simulink model "gm_qft_3qubit_fixpt"  (R2024b)
settings: Solver=VariableStepAuto  StartTime=0.0  StopTime=10.0  RelTol=1e-3
settings Model: SimulationMode=accelerator  Creator=bonga  LastModifiedBy=bonga
settings DebuggingCC: InheritedTsInSrcMsg=none

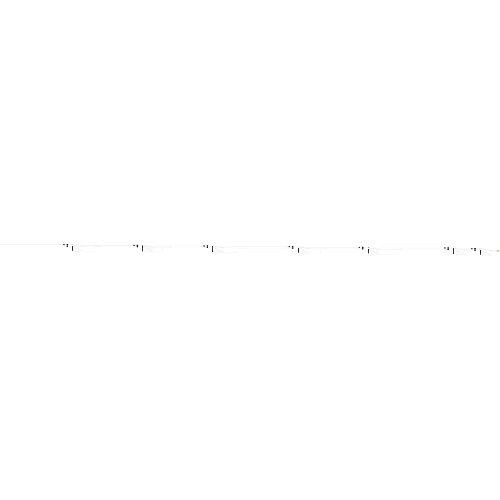
[thumbnail: Simulink's stored preview of the top-level diagram]
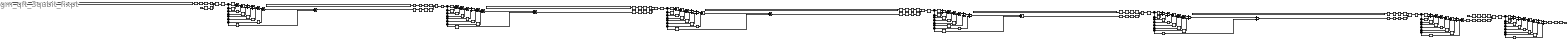
== system gm_qft_3qubit_fixpt ==
  initial_state : Inport  OutDataTypeStr=fixdt(0,1,0,'DataTypeOverride', 'Off')  PortDimensions=[8 1]  SampleTime=1
  MMul_add_01 : Sum  OutDataTypeStr=fixdt(1, 18, 14)  SampleTime=1
  MMul_add_011 : Sum  OutDataTypeStr=fixdt(1, 32, 26)  SampleTime=1
  MMul_add_012 : Sum  OutDataTypeStr=fixdt(1, 19, 13)  SampleTime=1
  MMul_add_013 : Sum  OutDataTypeStr=fixdt(1, 32, 26)  SampleTime=1
  MMul_add_014 : Sum  OutDataTypeStr=fixdt(1, 19, 13)  SampleTime=1
  MMul_add_015 : Sum  OutDataTypeStr=fixdt(1, 19, 13)  SampleTime=1
  MMul_add_016 : Sum  OutDataTypeStr=fixdt(1, 18, 13)  SampleTime=1
  MMul_add_{12,23,34,45,56,67} (6 alike) : Sum  OutDataTypeStr=fixdt(1, 18, 14)  SampleTime=1
  MMul_add_{121,123,231,233,341,343,451,453,561,563,671,673} (12 alike) : Sum  OutDataTypeStr=fixdt(1, 32, 26)  SampleTime=1
  MMul_add_{122,124..125,232,234..235,342,344..345,452,454..455,562,564..565,672,674..675} (18 alike) : Sum  OutDataTypeStr=fixdt(1, 19, 13)  SampleTime=1
  MMul_add_{126,236,346,456,566,676} (6 alike) : Sum  OutDataTypeStr=fixdt(1, 18, 13)  SampleTime=1
  MMul_dot_product : Product  Inputs=**  OutDataTypeStr=fixdt(1, 18, 14)  SampleTime=1
  MMul_dot_product1 : Product  Inputs=**  OutDataTypeStr=fixdt(1, 32, 26)  SampleTime=1
  MMul_dot_product2 : Product  Inputs=**  OutDataTypeStr=fixdt(1, 19, 13)  SampleTime=1
  MMul_dot_product3 : Product  Inputs=**  OutDataTypeStr=fixdt(1, 32, 26)  SampleTime=1
  MMul_dot_product4 : Product  Inputs=**  OutDataTypeStr=fixdt(1, 19, 13)  SampleTime=1
  MMul_dot_product5 : Product  Inputs=**  OutDataTypeStr=fixdt(1, 19, 13)  SampleTime=1
  MMul_dot_product6 : Product  Inputs=**  OutDataTypeStr=fixdt(1, 18, 13)  SampleTime=1
  Row2Col_in{0..1,11..16} (8 alike) : Reshape  OutputDimensionality=Column vector (2-D)
  Row2Col_in01 : Reshape  OutputDimensionality=Column vector (2-D)
  Row2Col_in02 : Reshape  OutputDimensionality=Column vector (2-D)
  Row2Col_in03 : Reshape  OutputDimensionality=Column vector (2-D)
  Row2Col_in04 : Reshape  OutputDimensionality=Column vector (2-D)
  Row2Col_in05 : Reshape  OutputDimensionality=Column vector (2-D)
  Row2Col_in06 : Reshape  OutputDimensionality=Column vector (2-D)
  dtc : DataTypeConversion  OutDataTypeStr=fixdt(1, 14, 14)  SampleTime=1  SaturateOnIntegerOverflow=off  RndMeth=Floor
  dtc1 : DataTypeConversion  OutDataTypeStr=fixdt(1, 14, 14)  SampleTime=1  SaturateOnIntegerOverflow=off  RndMeth=Floor
  dtc{2..7} (6 alike) : DataTypeConversion  OutDataTypeStr=fixdt(1, 14, 13)  SampleTime=1  SaturateOnIntegerOverflow=off  RndMeth=Floor
  final_state_reg : Delay  DelayLength=double(1)  InitialCondition=0  SampleTime=1
  gain_const : Constant  Value=[1;0;0;0;0;0;0;0;0;1;0;0;0;0;0;0;0;0;1;0;0;0;0;0;0;0;0;1;0;0;0;0;0;0;0;0;1;0;0;0;0;0;0;0;0;1;0;0;0;0;0;0;0;0;1;0;0;0;0;0;0;0;0;1]  OutDataTypeStr=fixdt(0, 1, 0)  SampleTime=1
  gain_const1 : Constant  Value="complex(fi(\"numerictype\",numerictype(1,14,13),\"fimath\",fimath(\"RoundingMethod\", \"Floor\",\"OverflowAction\", \"Wrap\",\"ProductMode\",\"FullPrecision\",\"SumMode\",\"FullPrecision\"),\"Value\",\"[0.70703125;0.70703125;0;0;0;0;0;0;0.70703125;-0.7071533203125;0;0;0;0;0;0;0;0;0.70703125;0.70703125;0;0;0;0;0;0;0.70703125;-0.7071533203125;0;0;0;0;0;0;0;0;0.70703125;0.70703125;0;0;0;0;0;0;0.70703125;-0.7071533203125;0;0;0;0;0;0;0;0;0.70703125;0.70703125;0;0;0;0;0;0;0.70703125;-0.7071533203125]\"), fi(\"numerictype\",numerictype(1,14,13),\"fimath\",fimath(\"RoundingMethod\", \"Floor\",\"OverflowAction\", \"Wrap\",\"ProductMode\",\"FullPrecision\",\"SumMode\",\"FullPrecision\"),\"Value\",\"[0;0;0;0;0;0;0;0;0;0;0;0;0;0;0;0;0;0;0;0;0;0;0;0;0;0;0;0;0;0;0;0;0;0;0;0;0;0;0;0;0;0;0;0;0;0;0;0;0;0;0;0;0;0;0;0;0;0;0;0;0;0;0;0]\"))"  OutDataTypeStr=fixdt(1, 14, 13)  SampleTime=1
  gain_const2 : Constant  Value="complex(fi(\"numerictype\",numerictype(0,1,0),\"fimath\",fimath(\"RoundingMethod\", \"Floor\",\"OverflowAction\", \"Wrap\",\"ProductMode\",\"FullPrecision\",\"SumMode\",\"FullPrecision\"),\"Value\",\"[1;0;0;0;0;0;0;0;0;1;0;0;0;0;0;0;0;0;1;0;0;0;0;0;0;0;0;1;0;0;0;0;0;0;0;0;1;0;0;0;0;0;0;0;0;1;0;0;0;0;0;0;0;0;1;0;0;0;0;0;0;0;0;1]\"), fi(\"numerictype\",numerictype(0,1,0),\"fimath\",fimath(\"RoundingMethod\", \"Floor\",\"OverflowAction\", \"Wrap\",\"ProductMode\",\"FullPrecision\",\"SumMode\",\"FullPrecision\"),\"Value\",\"[0;0;0;0;0;0;0;0;0;0;0;0;0;0;0;0;0;0;0;0;0;0;0;0;0;0;0;0;0;0;0;0;0;0;0;0;0;0;0;0;0;0;0;0;0;0;0;0;0;0;0;0;0;0;0;0;0;0;0;0;0;0;0;0]\"))"  OutDataTypeStr=fixdt(0, 1, 0)  SampleTime=1
  gain_const3 : Constant  Value="complex(fi(\"numerictype\",numerictype(1,14,13),\"fimath\",fimath(\"RoundingMethod\", \"Floor\",\"OverflowAction\", \"Wrap\",\"ProductMode\",\"FullPrecision\",\"SumMode\",\"FullPrecision\"),\"Value\",\"[0.70703125;0;0.70703125;0;0;0;0;0;0;0.70703125;0;0.70703125;0;0;0;0;0.70703125;0;-0.707275390625;0;0;0;0;0;0;0.70703125;0;-0.707275390625;0;0;0;0;0;0;0;0;0.70703125;0;0.70703125;0;0;0;0;0;0;0.70703125;0;0.70703125;0;0;0;0;0.70703125;0;-0.707275390625;0;0;0;0;0;0;0.70703125;0;-0.707275390625]\"), fi(\"numerictype\",numerictype(1,14,13),\"fimath\",fimath(\"RoundingMethod\", \"Floor\",\"OverflowAction\", \"Wrap\",\"ProductMode\",\"FullPrecision\",\"SumMode\",\"FullPrecision\"),\"Value\",\"[0;0;0;0;0;0;0;0;0;0;0;0;0;0;0;0;0;0;0;0;0;0;0;0;0;0;0;0;0;0;0;0;0;0;0;0;0;0;0;0;0;0;0;0;0;0;0;0;0;0;0;0;0;0;0;0;0;0;0;0;0;0;0;0]\"))"  OutDataTypeStr=fixdt(1, 14, 13)  SampleTime=1
  gain_const4 : Constant  Value="complex(fi(\"numerictype\",numerictype(0,1,0),\"fimath\",fimath(\"RoundingMethod\", \"Floor\",\"OverflowAction\", \"Wrap\",\"ProductMode\",\"FullPrecision\",\"SumMode\",\"FullPrecision\"),\"Value\",\"[1;0;0;0;0;0;0;0;0;1;0;0;0;0;0;0;0;0;1;0;0;0;0;0;0;0;0;1;0;0;0;0;0;0;0;0;1;0;0;0;0;0;0;0;0;1;0;0;0;0;0;0;0;0;1;0;0;0;0;0;0;0;0;1]\"), fi(\"numerictype\",numerictype(0,1,0),\"fimath\",fimath(\"RoundingMethod\", \"Floor\",\"OverflowAction\", \"Wrap\",\"ProductMode\",\"FullPrecision\",\"SumMode\",\"FullPrecision\"),\"Value\",\"[0;0;0;0;0;0;0;0;0;0;0;0;0;0;0;0;0;0;0;0;0;0;0;0;0;0;0;0;0;0;0;0;0;0;0;0;0;0;0;0;0;0;0;0;0;0;0;0;0;0;0;0;0;0;0;0;0;0;0;0;0;0;0;0]\"))"  OutDataTypeStr=fixdt(0, 1, 0)  SampleTime=1
  gain_const5 : Constant  Value="complex(fi(\"numerictype\",numerictype(0,1,0),\"fimath\",fimath(\"RoundingMethod\", \"Floor\",\"OverflowAction\", \"Wrap\",\"ProductMode\",\"FullPrecision\",\"SumMode\",\"FullPrecision\"),\"Value\",\"[1;0;0;0;0;0;0;0;0;1;0;0;0;0;0;0;0;0;1;0;0;0;0;0;0;0;0;1;0;0;0;0;0;0;0;0;1;0;0;0;0;0;0;0;0;1;0;0;0;0;0;0;0;0;1;0;0;0;0;0;0;0;0;1]\"), fi(\"numerictype\",numerictype(0,1,0),\"fimath\",fimath(\"RoundingMethod\", \"Floor\",\"OverflowAction\", \"Wrap\",\"ProductMode\",\"FullPrecision\",\"SumMode\",\"FullPrecision\"),\"Value\",\"[0;0;0;0;0;0;0;0;0;0;0;0;0;0;0;0;0;0;0;0;0;0;0;0;0;0;0;0;0;0;0;0;0;0;0;0;0;0;0;0;0;0;0;0;0;0;0;0;0;0;0;0;0;0;0;0;0;0;0;0;0;0;0;0]\"))"  OutDataTypeStr=fixdt(0, 1, 0)  SampleTime=1
  gain_const6 : Constant  Value="complex(fi(\"numerictype\",numerictype(1,14,13),\"fimath\",fimath(\"RoundingMethod\", \"Floor\",\"OverflowAction\", \"Wrap\",\"ProductMode\",\"FullPrecision\",\"SumMode\",\"FullPrecision\"),\"Value\",\"[0.70703125;0;0;0;0.70703125;0;0;0;0;0.70703125;0;0;0;0.70703125;0;0;0;0;0.70703125;0;0;0;0.70703125;0;0;0;0;0.70703125;0;0;0;0.70703125;0.70703125;0;0;0;-0.707275390625;0;0;0;0;0.70703125;0;0;0;-0.707275390625;0;0;0;0;0.70703125;0;0;0;-0.707275390625;0;0;0;0;0.70703125;0;0;0;-0.707275390625]\"), fi(\"numerictype\",numerictype(1,14,13),\"fimath\",fimath(\"RoundingMethod\", \"Floor\",\"OverflowAction\", \"Wrap\",\"ProductMode\",\"FullPrecision\",\"SumMode\",\"FullPrecision\"),\"Value\",\"[0;0;0;0;0;0;0;0;0;0;0;0;0;0;0;0;0;0;0;0;0;0;0;0;0;0;0;0;0;0;0;0;0;0;0;0;0;0;0;0;0;0;0;0;0;0;0;0;0;0;0;0;0;0;0;0;0;0;0;0;0;0;0;0]\"))"  OutDataTypeStr=fixdt(1, 14, 13)  SampleTime=1
  reshape_dotProduct{,1..6} (7 alike) : Reshape  OutputDimensionality=Customize  OutputDimensions=[8,8]
  reshape_mmulResult{,1..6} (7 alike) : Reshape  OutputDimensionality=Customize  OutputDimensions=[8,1]
  select_0 : Selector  NumberOfDimensions=2  IndexOptions=Index vector (dialog),Select all  Indices=double(1),[]  OutputSizes=1
  select_01 : Selector  NumberOfDimensions=2  IndexOptions=Index vector (dialog),Select all  Indices=double(1),[]  OutputSizes=1
  select_02 : Selector  NumberOfDimensions=2  IndexOptions=Index vector (dialog),Select all  Indices=double(1),[]  OutputSizes=1
  select_03 : Selector  NumberOfDimensions=2  IndexOptions=Index vector (dialog),Select all  Indices=double(1),[]  OutputSizes=1
  select_04 : Selector  NumberOfDimensions=2  IndexOptions=Index vector (dialog),Select all  Indices=double(1),[]  OutputSizes=1
  select_05 : Selector  NumberOfDimensions=2  IndexOptions=Index vector (dialog),Select all  Indices=double(1),[]  OutputSizes=1
  select_06 : Selector  NumberOfDimensions=2  IndexOptions=Index vector (dialog),Select all  Indices=double(1),[]  OutputSizes=1
  select_{1,11..16} (7 alike) : Selector  NumberOfDimensions=2  IndexOptions=Index vector (dialog),Select all  Indices=double(2),[]  OutputSizes=1
  select_{2,21..26} (7 alike) : Selector  NumberOfDimensions=2  IndexOptions=Index vector (dialog),Select all  Indices=double(3),[]  OutputSizes=1
  select_{3,31..36} (7 alike) : Selector  NumberOfDimensions=2  IndexOptions=Index vector (dialog),Select all  Indices=double(4),[]  OutputSizes=1
  select_{4,41..46} (7 alike) : Selector  NumberOfDimensions=2  IndexOptions=Index vector (dialog),Select all  Indices=double(5),[]  OutputSizes=1
  select_{5,51..56} (7 alike) : Selector  NumberOfDimensions=2  IndexOptions=Index vector (dialog),Select all  Indices=double(6),[]  OutputSizes=1
  select_{6,61..66} (7 alike) : Selector  NumberOfDimensions=2  IndexOptions=Index vector (dialog),Select all  Indices=double(7),[]  OutputSizes=1
  select_{7,71..76} (7 alike) : Selector  NumberOfDimensions=2  IndexOptions=Index vector (dialog),Select all  Indices=double(8),[]  OutputSizes=1
  select_indices0 : Selector  InputPortWidth=64  IndexOptions=Index vector (dialog)  Indices=double([1 9 17 25 33 41 49 57 2 10 18 26 34 42 50 58 3 11 19 27 35 43 51 59 4 12 20 28 36 44 52 60 5 13 21 29 37 45 53 61 6 14 22 30 38 46 54 62 7 15 23 31 39 47 55 63 8 16 24 32 40 48 56 64])  OutputSizes=1
  select_indices01 : Selector  InputPortWidth=64  IndexOptions=Index vector (dialog)  Indices=double([1 9 17 25 33 41 49 57 2 10 18 26 34 42 50 58 3 11 19 27 35 43 51 59 4 12 20 28 36 44 52 60 5 13 21 29 37 45 53 61 6 14 22 30 38 46 54 62 7 15 23 31 39 47 55 63 8 16 24 32 40 48 56 64])  OutputSizes=1
  select_indices02 : Selector  InputPortWidth=64  IndexOptions=Index vector (dialog)  Indices=double([1 9 17 25 33 41 49 57 2 10 18 26 34 42 50 58 3 11 19 27 35 43 51 59 4 12 20 28 36 44 52 60 5 13 21 29 37 45 53 61 6 14 22 30 38 46 54 62 7 15 23 31 39 47 55 63 8 16 24 32 40 48 56 64])  OutputSizes=1
  select_indices03 : Selector  InputPortWidth=64  IndexOptions=Index vector (dialog)  Indices=double([1 9 17 25 33 41 49 57 2 10 18 26 34 42 50 58 3 11 19 27 35 43 51 59 4 12 20 28 36 44 52 60 5 13 21 29 37 45 53 61 6 14 22 30 38 46 54 62 7 15 23 31 39 47 55 63 8 16 24 32 40 48 56 64])  OutputSizes=1
  select_indices04 : Selector  InputPortWidth=64  IndexOptions=Index vector (dialog)  Indices=double([1 9 17 25 33 41 49 57 2 10 18 26 34 42 50 58 3 11 19 27 35 43 51 59 4 12 20 28 36 44 52 60 5 13 21 29 37 45 53 61 6 14 22 30 38 46 54 62 7 15 23 31 39 47 55 63 8 16 24 32 40 48 56 64])  OutputSizes=1
  select_indices05 : Selector  InputPortWidth=64  IndexOptions=Index vector (dialog)  Indices=double([1 9 17 25 33 41 49 57 2 10 18 26 34 42 50 58 3 11 19 27 35 43 51 59 4 12 20 28 36 44 52 60 5 13 21 29 37 45 53 61 6 14 22 30 38 46 54 62 7 15 23 31 39 47 55 63 8 16 24 32 40 48 56 64])  OutputSizes=1
  select_indices06 : Selector  InputPortWidth=64  IndexOptions=Index vector (dialog)  Indices=double([1 9 17 25 33 41 49 57 2 10 18 26 34 42 50 58 3 11 19 27 35 43 51 59 4 12 20 28 36 44 52 60 5 13 21 29 37 45 53 61 6 14 22 30 38 46 54 62 7 15 23 31 39 47 55 63 8 16 24 32 40 48 56 64])  OutputSizes=1
  select_indices{1,11..16} (7 alike) : Selector  InputPortWidth=8  IndexOptions=Index vector (dialog)  Indices=double([1 2 3 4 5 6 7 8 1 2 3 4 5 6 7 8 1 2 3 4 5 6 7 8 1 2 3 4 5 6 7 8 1 2 3 4 5 6 7 8 1 2 3 4 5 6 7 8 1 2 3 4 5 6 7 8 1 2 3 4 5 6 7 8])  OutputSizes=1
  t{,1..6} (7 alike) : Reshape  OutputDimensionality=Customize  OutputDimensions=[8,8]
  vectorized_in0 : Reshape  OutputDimensionality=Row vector (2-D)
  vectorized_in01 : Reshape  OutputDimensionality=Row vector (2-D)
  vectorized_in02 : Reshape  OutputDimensionality=Row vector (2-D)
  vectorized_in03 : Reshape  OutputDimensionality=Row vector (2-D)
  vectorized_in04 : Reshape  OutputDimensionality=Row vector (2-D)
  vectorized_in05 : Reshape  OutputDimensionality=Row vector (2-D)
  vectorized_in06 : Reshape  OutputDimensionality=Row vector (2-D)
  final_state : Outport  OutDataTypeStr=fixdt(1,14,14,'DataTypeOverride', 'Off')  PortDimensions=[8 1]  SampleTime=1
      settings: SignalType=complex
  wires:
  select_indices0/1 -> Row2Col_in0/1
  dtc2/1 -> dtc1/1
  gain_const4/1 -> t4/1
  select_01/1 -> MMul_add_011/1
  reshape_mmulResult1/1 -> dtc2/1
  select_0/1 -> MMul_add_01/1
  MMul_add_561/1 -> MMul_add_671/1
  reshape_mmulResult2/1 -> dtc3/1
  reshape_mmulResult3/1 -> dtc4/1
  dtc6/1 -> select_indices14/1
  select_indices01/1 -> Row2Col_in01/1
  reshape_mmulResult5/1 -> dtc6/1
  dtc7/1 -> select_indices15/1
  select_indices1/1 -> Row2Col_in1/1
  vectorized_in0/1 -> select_indices0/1
  Row2Col_in0/1 -> MMul_dot_product/1
  MMul_dot_product/1 -> reshape_dotProduct/1
  select_12/1 -> MMul_add_012/2
  MMul_add_12/1 -> MMul_add_23/1
  select_4/1 -> MMul_add_34/2
  select_5/1 -> MMul_add_45/2
  select_53/1 -> MMul_add_453/2
  t1/1 -> vectorized_in01/1
  MMul_add_011/1 -> MMul_add_121/1
  MMul_add_673/1 -> reshape_mmulResult3/1
  MMul_add_234/1 -> MMul_add_344/1
  MMul_add_344/1 -> MMul_add_454/1
  t5/1 -> vectorized_in05/1
  MMul_add_564/1 -> MMul_add_674/1
  MMul_add_34/1 -> MMul_add_45/1
  select_11/1 -> MMul_add_011/2
  select_15/1 -> MMul_add_015/2
  select_16/1 -> MMul_add_016/2
  select_54/1 -> MMul_add_454/2
  select_63/1 -> MMul_add_563/2
  MMul_add_015/1 -> MMul_add_125/1
  select_64/1 -> MMul_add_564/2
  select_24/1 -> MMul_add_124/2
  MMul_add_235/1 -> MMul_add_345/1
  MMul_add_236/1 -> MMul_add_346/1
  MMul_add_125/1 -> MMul_add_235/1
  gain_const3/1 -> t3/1
  select_43/1 -> MMul_add_343/2
  MMul_add_676/1 -> reshape_mmulResult6/1
  select_26/1 -> MMul_add_126/2
  select_indices14/1 -> Row2Col_in14/1
  gain_const2/1 -> t2/1
  vectorized_in03/1 -> select_indices03/1
  MMul_add_121/1 -> MMul_add_231/1
  reshape_dotProduct6/1 -> select_76/1, select_66/1, select_56/1, select_46/1, select_36/1, select_26/1, select_16/1, select_06/1
  reshape_mmulResult4/1 -> dtc5/1
  reshape_dotProduct4/1 -> select_74/1, select_64/1, select_54/1, select_44/1, select_34/1, select_24/1, select_14/1, select_04/1
  select_indices13/1 -> Row2Col_in13/1
  select_indices11/1 -> Row2Col_in11/1
  select_14/1 -> MMul_add_014/2
  select_21/1 -> MMul_add_121/2
  MMul_add_671/1 -> reshape_mmulResult1/1
  MMul_dot_product1/1 -> reshape_dotProduct1/1
  select_04/1 -> MMul_add_014/1
  Row2Col_in13/1 -> MMul_dot_product3/2
  select_73/1 -> MMul_add_673/2
  select_indices16/1 -> Row2Col_in16/1
  dtc4/1 -> select_indices12/1
  select_06/1 -> MMul_add_016/1
  select_75/1 -> MMul_add_675/2
  Row2Col_in03/1 -> MMul_dot_product3/1
  select_indices04/1 -> Row2Col_in04/1
  MMul_add_122/1 -> MMul_add_232/1
  select_7/1 -> MMul_add_67/2
  MMul_add_123/1 -> MMul_add_233/1
  MMul_add_231/1 -> MMul_add_341/1
  select_42/1 -> MMul_add_342/2
  Row2Col_in15/1 -> MMul_dot_product5/2
  reshape_dotProduct2/1 -> select_62/1, select_72/1, select_52/1, select_42/1, select_32/1, select_22/1, select_12/1, select_02/1
  select_02/1 -> MMul_add_012/1
  select_62/1 -> MMul_add_562/2
  gain_const6/1 -> t6/1
  select_indices06/1 -> Row2Col_in06/1
  vectorized_in05/1 -> select_indices05/1
  t4/1 -> vectorized_in04/1
  MMul_add_342/1 -> MMul_add_452/1
  t3/1 -> vectorized_in03/1
  MMul_dot_product4/1 -> reshape_dotProduct4/1
  vectorized_in02/1 -> select_indices02/1
  select_41/1 -> MMul_add_341/2
  Row2Col_in01/1 -> MMul_dot_product1/1
  select_22/1 -> MMul_add_122/2
  select_34/1 -> MMul_add_234/2
  Row2Col_in12/1 -> MMul_dot_product2/2
  MMul_add_343/1 -> MMul_add_453/1
  MMul_add_562/1 -> MMul_add_672/1
  t/1 -> vectorized_in0/1
  MMul_add_01/1 -> MMul_add_12/1
  vectorized_in01/1 -> select_indices01/1
  select_03/1 -> MMul_add_013/1
  select_32/1 -> MMul_add_232/2
  MMul_add_233/1 -> MMul_add_343/1
  select_2/1 -> MMul_add_12/2
  MMul_add_453/1 -> MMul_add_563/1
  dtc5/1 -> select_indices13/1
  MMul_add_346/1 -> MMul_add_456/1
  MMul_dot_product3/1 -> reshape_dotProduct3/1
  reshape_dotProduct1/1 -> select_71/1, select_61/1, select_51/1, select_41/1, select_31/1, select_21/1, select_11/1, select_01/1
  MMul_add_23/1 -> MMul_add_34/1
  gain_const5/1 -> t5/1
  gain_const1/1 -> t1/1
  MMul_add_452/1 -> MMul_add_562/1
  select_72/1 -> MMul_add_672/2
  select_46/1 -> MMul_add_346/2
  MMul_add_451/1 -> MMul_add_561/1
  Row2Col_in04/1 -> MMul_dot_product4/1
  select_61/1 -> MMul_add_561/2
  MMul_add_232/1 -> MMul_add_342/1
  reshape_mmulResult/1 -> dtc/1
  vectorized_in04/1 -> select_indices04/1
  select_05/1 -> MMul_add_015/1
  MMul_add_013/1 -> MMul_add_123/1
  select_45/1 -> MMul_add_345/2
  select_66/1 -> MMul_add_566/2
  select_13/1 -> MMul_add_013/2
  dtc1/1 -> select_indices1/1
  MMul_add_563/1 -> MMul_add_673/1
  Row2Col_in05/1 -> MMul_dot_product5/1
  select_44/1 -> MMul_add_344/2
  Row2Col_in11/1 -> MMul_dot_product1/2
  MMul_add_675/1 -> reshape_mmulResult5/1
  dtc3/1 -> select_indices11/1
  MMul_dot_product2/1 -> reshape_dotProduct2/1
  select_74/1 -> MMul_add_674/2
  select_33/1 -> MMul_add_233/2
  t2/1 -> vectorized_in02/1
  MMul_add_124/1 -> MMul_add_234/1
  Row2Col_in14/1 -> MMul_dot_product4/2
  Row2Col_in16/1 -> MMul_dot_product6/2
  MMul_add_456/1 -> MMul_add_566/1
  select_indices12/1 -> Row2Col_in12/1
  MMul_add_674/1 -> reshape_mmulResult4/1
  select_indices02/1 -> Row2Col_in02/1
  select_indices03/1 -> Row2Col_in03/1
  MMul_dot_product5/1 -> reshape_dotProduct5/1
  reshape_mmulResult6/1 -> dtc7/1
  select_31/1 -> MMul_add_231/2
  MMul_add_341/1 -> MMul_add_451/1
  MMul_dot_product6/1 -> reshape_dotProduct6/1
  select_52/1 -> MMul_add_452/2
  MMul_add_016/1 -> MMul_add_126/1
  select_76/1 -> MMul_add_676/2
  reshape_dotProduct5/1 -> select_65/1, select_75/1, select_55/1, select_45/1, select_35/1, select_25/1, select_15/1, select_05/1
  MMul_add_012/1 -> MMul_add_122/1
  select_6/1 -> MMul_add_56/2
  t6/1 -> vectorized_in06/1
  MMul_add_566/1 -> MMul_add_676/1
  Row2Col_in02/1 -> MMul_dot_product2/1
  MMul_add_565/1 -> MMul_add_675/1
  select_3/1 -> MMul_add_23/2
  MMul_add_454/1 -> MMul_add_564/1
  dtc/1 -> final_state_reg/1
  MMul_add_45/1 -> MMul_add_56/1
  select_56/1 -> MMul_add_456/2
  select_35/1 -> MMul_add_235/2
  final_state_reg/1 -> final_state/1
  select_25/1 -> MMul_add_125/2
  MMul_add_672/1 -> reshape_mmulResult2/1
  Row2Col_in1/1 -> MMul_dot_product/2
  MMul_add_014/1 -> MMul_add_124/1
  reshape_dotProduct/1 -> select_7/1, select_6/1, select_5/1, select_4/1, select_3/1, select_2/1, select_1/1, select_0/1
  MMul_add_67/1 -> reshape_mmulResult/1
  vectorized_in06/1 -> select_indices06/1
  select_23/1 -> MMul_add_123/2
  Row2Col_in06/1 -> MMul_dot_product6/1
  MMul_add_56/1 -> MMul_add_67/1
  select_65/1 -> MMul_add_565/2
  select_1/1 -> MMul_add_01/2
  reshape_dotProduct3/1 -> select_73/1, select_63/1, select_53/1, select_43/1, select_33/1, select_23/1, select_13/1, select_03/1
  select_55/1 -> MMul_add_455/2
  gain_const/1 -> t/1
  select_indices15/1 -> Row2Col_in15/1
  MMul_add_345/1 -> MMul_add_455/1
  initial_state/1 -> select_indices16/1
  select_indices05/1 -> Row2Col_in05/1
  select_51/1 -> MMul_add_451/2
  MMul_add_126/1 -> MMul_add_236/1
  select_71/1 -> MMul_add_671/2
  select_36/1 -> MMul_add_236/2
  MMul_add_455/1 -> MMul_add_565/1
